simulink model "lab02"  (Simulink 9.2)
settings: Solver=ode45  StartTime=0.0  StopTime=0.312  RelTol=1e-3  EnableMultiTasking=on
values from neighbouring files (symbols this model uses):
  Ja = 0.000036    (= 3.6e-05)    [Func_L_2.m]    (also in lab02.m)
  Ke = 0.057    [Func_L_2.m]    (also in lab02.m)
  Km = 0.057    [Func_L_2.m]    (also in lab02.m)
  La = 0.004    [Func_L_2.m]    (also in lab02.m)
  M = Mnom*2*i1/(Nm-1); M1(i)=M    [Func_L_2.m]    (also in lab02.m)
  Ra = 4.0    (= 4)    [Func_L_2.m]    (also in lab02.m)
  U = Unom*2*j1/(Nu-1); U1(j)=U    [Func_L_2.m]    (also in lab02.m)
settings Model: Creator=PC  LastModifiedBy=murad  ExtModeTrigMode=oneshot  ExtModeArmWhenConnect=off
settings DataIOCC: LimitDataPoints=off  SignalLoggingName=sigsOut
settings OptimizationCC: BooleanDataType=off  LifeSpan=auto
settings DebuggingCC: SaveWithParameterizedLinksMsg=none  SignalResolutionControl=TryResolveAllWithWarning  MultiTaskDSMMsg=warning  MultiTaskCondExecSysMsg=none  FcnCallInpInsideContextMsg=error  StateNameClashWarn=none  SFUnexpectedBacktrackingDiag=error  SFNoUnconditionalDefaultTransitionDiag=error  SFExecutionAtInitializationDiag=warning
settings HardwareCC: TargetUnknown=on
settings SFSimCC: SimUseLocalCustomCode=on
settings RTWCC: RTWUseLocalCustomCode=on
settings CodeAppCC: StateflowObjectComments=off
settings GRTTargetCC: TargetLangStandard=C99 (ISO)  GeneratePreprocessorConditionals=Use local settings
settings ConfigComp: CovExternalEMLEnable=on

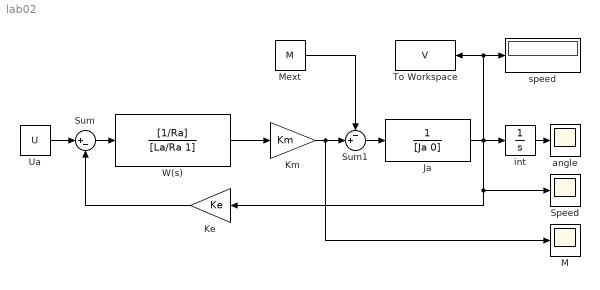
== system lab02 ==
  Ja : TransferFcn  Denominator=[Ja 0]
  Ke : Gain  Gain=Ke  SaturateOnIntegerOverflow=on  OutDataTypeStr=Inherit: Same as input  ParamDataTypeStr=Inherit: Same as input
  Km : Gain  Gain=Km  SaturateOnIntegerOverflow=on  OutDataTypeStr=Inherit: Same as input  ParamDataTypeStr=Inherit: Same as input
  M : Scope
  Mext : Constant  Value=M
  Speed : Scope
  Sum : Sum  Inputs=|+-  SaturateOnIntegerOverflow=on  InputSameDT=on  OutDataTypeStr=Inherit: Same as first input
  Sum1 : Sum  Inputs=-+|  SaturateOnIntegerOverflow=on  InputSameDT=on  OutDataTypeStr=Inherit: Same as first input
  To Workspace : ToWorkspace  VariableName=V  SampleTime=-1
  Ua : Constant  Value=U
  W(s) : TransferFcn  Numerator=[1/Ra]  Denominator=[La/Ra 1]
  angle : Scope
  int : Integrator
  speed : Display
  wires:
  Sum/1 -> W(s)/1
  W(s)/1 -> Km/1
  Mext/1 -> Sum1/1
  Ke/1 -> Sum/2
  Sum1/1 -> Ja/1
  Ja/1 -> int/1, Ke/1, Speed/1, To Workspace/1, speed/1
  int/1 -> angle/1
  Km/1 -> M/1, Sum1/2
  Ua/1 -> Sum/1
